simulink model "right_hand_rule"  (R2016a)
settings: Solver=FixedStepAuto  StartTime=0.0  StopTime=10.0  FixedStep=0.002  RelTol=1e-3
undefined symbols (not defined in the file or in its folder): exterm
libraries: simulink x1
settings Model: Creator=max  LastModifiedBy=max

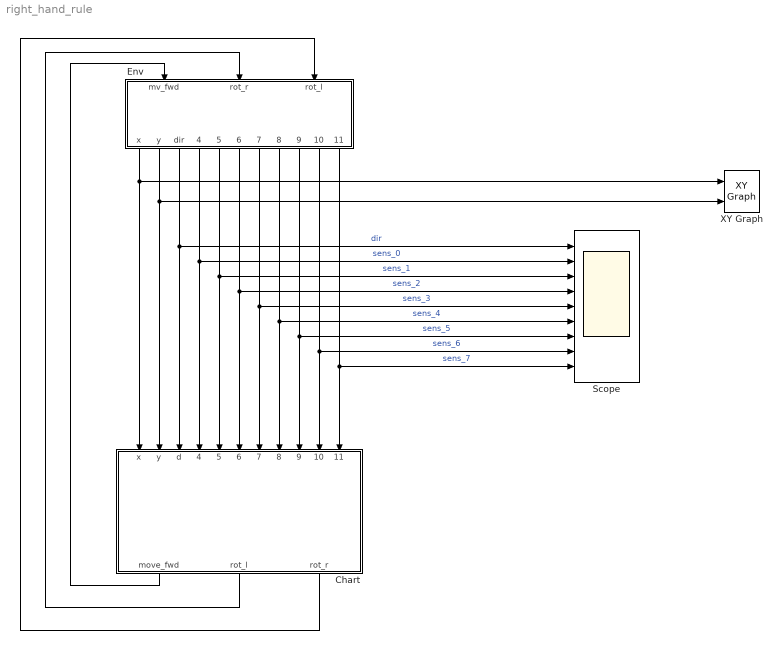
== system right_hand_rule ==
  Chart : Stateflow chart  TreatAsAtomicUnit=on
  Env : Subsystem
  Scope : Scope  NumInputPorts=9
  XY Graph : simulink/Sinks/XY Graph  xmin=-1  xmax=1  ymin=-1  ymax=1  st=-1
  wires:
  Chart/1(move_fwd) -> Env/1(mv_fwd)
  Chart/2(rot_l) -> Env/2(rot_r)
  Chart/3(rot_r) -> Env/3(rot_l)
  Env/1(x) -> Chart/1(x), XY Graph/1
  Env/4(sens_0) -> Chart/4(s_m150), Scope/2  "sens_0"
  Env/5(sens_1) -> Chart/5(s_m90), Scope/3  "sens_1"
  Env/6(sens_2) -> Chart/6(s_m45), Scope/4  "sens_2"
  Env/7(sens_3) -> Chart/7(s_m20), Scope/5  "sens_3"
  Env/8(sens_4) -> Chart/8(s_p20), Scope/6  "sens_4"
  Env/9(sens_5) -> Chart/9(s_p45), Scope/7  "sens_5"
  Env/10(sens_6) -> Chart/10(s_p90), Scope/8  "sens_6"
  Env/11(sens_7) -> Chart/11(s_p150), Scope/9  "sens_7"
  Env/2(y) -> Chart/2(y), XY Graph/2
  Env/3(dir) -> Chart/3(d), Scope/1  "dir"

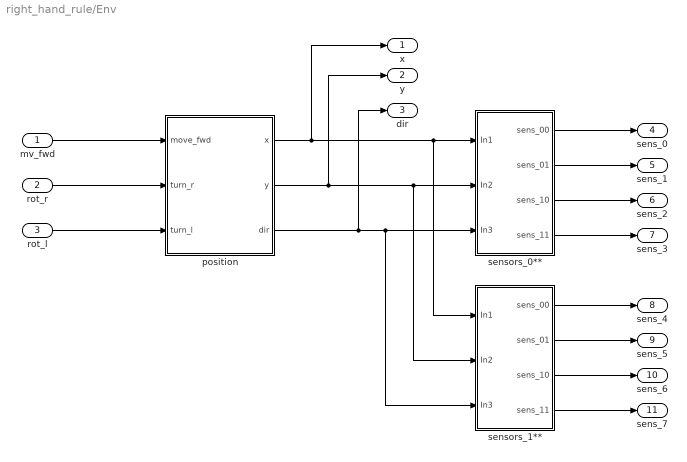
== system right_hand_rule/Env ==
  mv_fwd : Inport
  rot_r : Inport  Port=2
  rot_l : Inport  Port=3
  position : Subsystem
  sensors_0** : Subsystem
  sensors_1** : Subsystem
  x : Outport
  y : Outport  Port=2
  dir : Outport  Port=3
  sens_0 : Outport  Port=4
  sens_1 : Outport  Port=5
  sens_2 : Outport  Port=6
  sens_3 : Outport  Port=7
  sens_4 : Outport  Port=8
  sens_5 : Outport  Port=9
  sens_6 : Outport  Port=10
  sens_7 : Outport  Port=11
  wires:
  mv_fwd/1 -> position/1(move_fwd)
  rot_r/1 -> position/2(turn_r)
  rot_l/1 -> position/3(turn_l)
  sensors_0**/1(sens_00) -> sens_0/1
  sensors_0**/2(sens_01) -> sens_1/1
  sensors_0**/3(sens_10) -> sens_2/1
  sensors_0**/4(sens_11) -> sens_3/1
  position/1(x) -> x/1, sensors_1**/1(In1), sensors_0**/1(In1)
  position/2(y) -> sensors_1**/2(In2), sensors_0**/2(In2), y/1
  position/3(dir) -> dir/1, sensors_1**/3(In3), sensors_0**/3(In3)
  sensors_1**/1(sens_00) -> sens_4/1
  sensors_1**/2(sens_01) -> sens_5/1
  sensors_1**/3(sens_10) -> sens_6/1
  sensors_1**/4(sens_11) -> sens_7/1

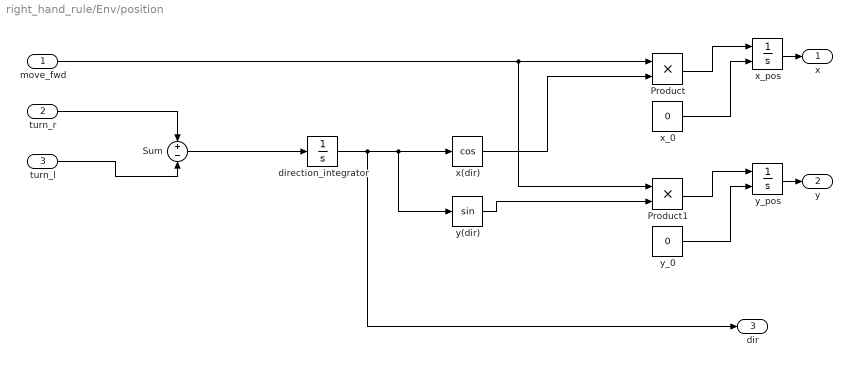
== system right_hand_rule/Env/position ==
  move_fwd : Inport
  turn_r : Inport  Port=2
  turn_l : Inport  Port=3
  Product : Product
  Product1 : Product
  Sum : Sum  Inputs=+-
  "direction_integrator " : Integrator
  x(dir) : Trigonometry  Operator=cos
  x_0 : Constant  Value=0
  x_pos : Integrator  InitialConditionSource=external  InitialCondition=exterm
  y(dir) : Trigonometry
  y_0 : Constant  Value=0
  y_pos : Integrator  InitialConditionSource=external  InitialCondition=exterm
  x : Outport
  y : Outport  Port=2
  dir : Outport  Port=3
  wires:
  turn_l/1 -> Sum/2
  Sum/1 -> "direction_integrator "/1
  turn_r/1 -> Sum/1
  y_pos/1 -> y/1
  x_0/1 -> x_pos/2
  x_pos/1 -> x/1
  x(dir)/1 -> Product/2
  Product/1 -> x_pos/1
  y(dir)/1 -> Product1/2
  Product1/1 -> y_pos/1
  move_fwd/1 -> Product1/1, Product/1
  y_0/1 -> y_pos/2
  "direction_integrator "/1 -> dir/1, y(dir)/1, x(dir)/1

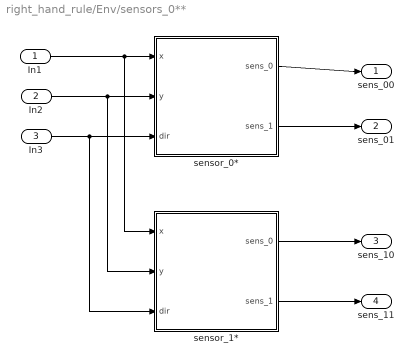
== system right_hand_rule/Env/sensors_0** ==
  In1 : Inport
  In2 : Inport  Port=2
  In3 : Inport  Port=3
  sensor_0* : Subsystem
  sensor_1* : Subsystem
  sens_00 : Outport
  sens_01 : Outport  Port=2
  sens_10 : Outport  Port=3
  sens_11 : Outport  Port=4
  wires:
  In3/1 -> sensor_1*/3(dir), sensor_0*/3(dir)
  sensor_1*/1(sens_0) -> sens_10/1
  sensor_1*/2(sens_1) -> sens_11/1
  sensor_0*/1(sens_0) -> sens_00/1
  sensor_0*/2(sens_1) -> sens_01/1
  In2/1 -> sensor_1*/2(y), sensor_0*/2(y)
  In1/1 -> sensor_1*/1(x), sensor_0*/1(x)

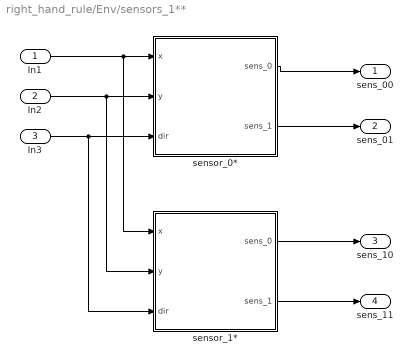
== system right_hand_rule/Env/sensors_1** ==
  In1 : Inport
  In2 : Inport  Port=2
  In3 : Inport  Port=3
  sensor_0* : Subsystem
  sensor_1* : Subsystem
  sens_00 : Outport
  sens_01 : Outport  Port=2
  sens_10 : Outport  Port=3
  sens_11 : Outport  Port=4
  wires:
  In3/1 -> sensor_1*/3(dir), sensor_0*/3(dir)
  sensor_1*/1(sens_0) -> sens_10/1
  sensor_1*/2(sens_1) -> sens_11/1
  sensor_0*/1(sens_0) -> sens_00/1
  sensor_0*/2(sens_1) -> sens_01/1
  In2/1 -> sensor_1*/2(y), sensor_0*/2(y)
  In1/1 -> sensor_1*/1(x), sensor_0*/1(x)

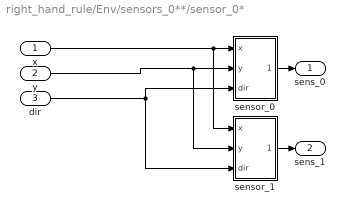
== system right_hand_rule/Env/sensors_0**/sensor_0* ==
  x : Inport
  y : Inport  Port=2
  dir : Inport  Port=3
  sensor_0 : Subsystem
  sensor_1 : Subsystem
  sens_0 : Outport
  sens_1 : Outport  Port=2
  wires:
  y/1 -> sensor_1/2(y), sensor_0/2(y)
  x/1 -> sensor_1/1(x), sensor_0/1(x)
  dir/1 -> sensor_1/3(dir), sensor_0/3(dir)
  sensor_0/1(dist) -> sens_0/1
  sensor_1/1(dist) -> sens_1/1

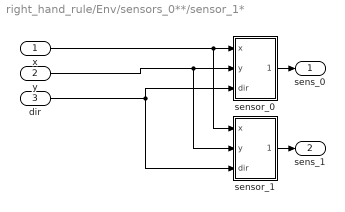
== system right_hand_rule/Env/sensors_0**/sensor_1* ==
  x : Inport
  y : Inport  Port=2
  dir : Inport  Port=3
  sensor_0 : Subsystem
  sensor_1 : Subsystem
  sens_0 : Outport
  sens_1 : Outport  Port=2
  wires:
  y/1 -> sensor_1/2(y), sensor_0/2(y)
  x/1 -> sensor_1/1(x), sensor_0/1(x)
  dir/1 -> sensor_1/3(dir), sensor_0/3(dir)
  sensor_0/1(dist) -> sens_0/1
  sensor_1/1(dist) -> sens_1/1

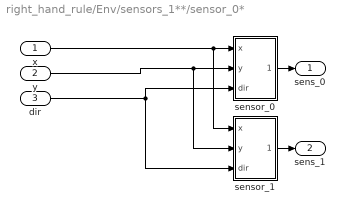
== system right_hand_rule/Env/sensors_1**/sensor_0* ==
  x : Inport
  y : Inport  Port=2
  dir : Inport  Port=3
  sensor_0 : Subsystem
  sensor_1 : Subsystem
  sens_0 : Outport
  sens_1 : Outport  Port=2
  wires:
  y/1 -> sensor_1/2(y), sensor_0/2(y)
  x/1 -> sensor_1/1(x), sensor_0/1(x)
  dir/1 -> sensor_1/3(dir), sensor_0/3(dir)
  sensor_0/1(dist) -> sens_0/1
  sensor_1/1(dist) -> sens_1/1

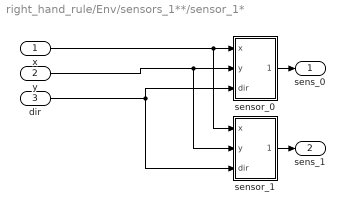
== system right_hand_rule/Env/sensors_1**/sensor_1* ==
  x : Inport
  y : Inport  Port=2
  dir : Inport  Port=3
  sensor_0 : Subsystem
  sensor_1 : Subsystem
  sens_0 : Outport
  sens_1 : Outport  Port=2
  wires:
  y/1 -> sensor_1/2(y), sensor_0/2(y)
  x/1 -> sensor_1/1(x), sensor_0/1(x)
  dir/1 -> sensor_1/3(dir), sensor_0/3(dir)
  sensor_0/1(dist) -> sens_0/1
  sensor_1/1(dist) -> sens_1/1

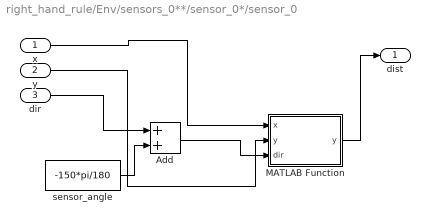
== system right_hand_rule/Env/sensors_0**/sensor_0*/sensor_0 ==
  x : Inport
  y : Inport  Port=2
  dir : Inport  Port=3
  Add : Sum
  MATLAB Function : MATLAB Function  TreatAsAtomicUnit=on
  sensor_angle : Constant  Value=-150*pi/180
  dist : Outport
  wires:
  sensor_angle/1 -> Add/2
  MATLAB Function/1(y) -> dist/1
  dir/1 -> Add/1
  Add/1 -> MATLAB Function/3(dir)
  x/1 -> MATLAB Function/1(x)
  y/1 -> MATLAB Function/2("y ")

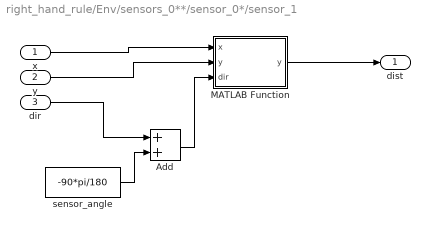
== system right_hand_rule/Env/sensors_0**/sensor_0*/sensor_1 ==
  x : Inport
  y : Inport  Port=2
  dir : Inport  Port=3
  Add : Sum
  MATLAB Function : MATLAB Function  TreatAsAtomicUnit=on
  sensor_angle : Constant  Value=-90*pi/180
  dist : Outport
  wires:
  sensor_angle/1 -> Add/2
  MATLAB Function/1(y) -> dist/1
  dir/1 -> Add/1
  Add/1 -> MATLAB Function/3(dir)
  x/1 -> MATLAB Function/1(x)
  y/1 -> MATLAB Function/2("y ")

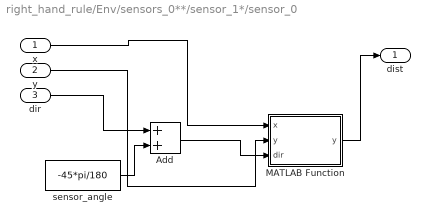
== system right_hand_rule/Env/sensors_0**/sensor_1*/sensor_0 ==
  x : Inport
  y : Inport  Port=2
  dir : Inport  Port=3
  Add : Sum
  MATLAB Function : MATLAB Function  TreatAsAtomicUnit=on
  sensor_angle : Constant  Value=-45*pi/180
  dist : Outport
  wires:
  sensor_angle/1 -> Add/2
  MATLAB Function/1(y) -> dist/1
  dir/1 -> Add/1
  Add/1 -> MATLAB Function/3(dir)
  x/1 -> MATLAB Function/1(x)
  y/1 -> MATLAB Function/2("y ")

== system right_hand_rule/Env/sensors_0**/sensor_1*/sensor_1 ==
  x : Inport
  y : Inport  Port=2
  dir : Inport  Port=3
  Add : Sum
  MATLAB Function : MATLAB Function  TreatAsAtomicUnit=on
  sensor_angle : Constant  Value=-20*pi/180
  dist : Outport
  wires:
  sensor_angle/1 -> Add/2
  MATLAB Function/1(y) -> dist/1
  dir/1 -> Add/1
  Add/1 -> MATLAB Function/3(dir)
  x/1 -> MATLAB Function/1(x)
  y/1 -> MATLAB Function/2("y ")

== system right_hand_rule/Env/sensors_1**/sensor_0*/sensor_0 ==
  x : Inport
  y : Inport  Port=2
  dir : Inport  Port=3
  Add : Sum
  MATLAB Function : MATLAB Function  TreatAsAtomicUnit=on
  sensor_angle : Constant  Value=20*pi/180
  dist : Outport
  wires:
  sensor_angle/1 -> Add/2
  MATLAB Function/1(y) -> dist/1
  dir/1 -> Add/1
  Add/1 -> MATLAB Function/3(dir)
  x/1 -> MATLAB Function/1(x)
  y/1 -> MATLAB Function/2("y ")

== system right_hand_rule/Env/sensors_1**/sensor_0*/sensor_1 ==
  x : Inport
  y : Inport  Port=2
  dir : Inport  Port=3
  Add : Sum
  MATLAB Function : MATLAB Function  TreatAsAtomicUnit=on
  sensor_angle : Constant  Value=45*pi/180
  dist : Outport
  wires:
  sensor_angle/1 -> Add/2
  MATLAB Function/1(y) -> dist/1
  dir/1 -> Add/1
  Add/1 -> MATLAB Function/3(dir)
  x/1 -> MATLAB Function/1(x)
  y/1 -> MATLAB Function/2("y ")

== system right_hand_rule/Env/sensors_1**/sensor_1*/sensor_0 ==
  x : Inport
  y : Inport  Port=2
  dir : Inport  Port=3
  Add : Sum
  MATLAB Function : MATLAB Function  TreatAsAtomicUnit=on
  sensor_angle : Constant  Value=90*pi/180
  dist : Outport
  wires:
  sensor_angle/1 -> Add/2
  MATLAB Function/1(y) -> dist/1
  dir/1 -> Add/1
  Add/1 -> MATLAB Function/3(dir)
  x/1 -> MATLAB Function/1(x)
  y/1 -> MATLAB Function/2("y ")

== system right_hand_rule/Env/sensors_1**/sensor_1*/sensor_1 ==
  x : Inport
  y : Inport  Port=2
  dir : Inport  Port=3
  Add : Sum
  MATLAB Function : MATLAB Function  TreatAsAtomicUnit=on
  sensor_angle : Constant  Value=150*pi/180
  dist : Outport
  wires:
  sensor_angle/1 -> Add/2
  MATLAB Function/1(y) -> dist/1
  dir/1 -> Add/1
  Add/1 -> MATLAB Function/3(dir)
  x/1 -> MATLAB Function/1(x)
  y/1 -> MATLAB Function/2("y ")

== matlab function right_hand_rule/Env/sensors_0**/sensor_0*/sensor_1/MATLAB Function ==
  data: x input; y output; y input; dir input
function y = fcn(x,y,dir)
y = intersectQuarterPlane(x,y,dir);

== matlab function right_hand_rule/Env/sensors_0**/sensor_0*/sensor_0/MATLAB Function ==
  data: x input; y output; y input; dir input
function y = fcn(x,y,dir)
y = intersectQuarterPlane(x,y,dir);

== stateflow chart right_hand_rule/Chart ==
  state claustrophobia
    % known: have -20, -45, -90
    entry:
    move_fwd = 0;
    rot_l = 1;
    rot_r = 0;
  state avoidCollision
    % known: have -20, -45
    entry:
    move_fwd = 0;
    rot_l = 1;
    rot_r = 0;
  state orientToWall
    % known: have -20
    % rotate left until we "touch the wall"
    entry:
    move_fwd = 1;
    rot_r = 0;
    rot_l = 0;
  state findWall
    entry:
    move_fwd=1;
    rot_l = d + 0;
    rot_r = 0;
  state follow
    % known: have -45, -90
    entry:
    move_fwd = 1;
    rot_l = 0;
    rot_r = 0;
  state stayClose
    % known: have -90, NOT have -45
    entry:
    move_fwd = 0;
    rot_l = 0;
    rot_r = 1;
  (default) -> findWall
  orientToWall -> avoidCollision : [s_m45 <= sens_tol]
  avoidCollision -> claustrophobia [order 2] : [s_m90 <= sens_tol]
  avoidCollision -> orientToWall [order 1] : [s_m45 > sens_tol]
  findWall -> orientToWall : [s_m20 <= sens_tol]
  stayClose -> orientToWall : [s_m20 <= sens_tol && after(90*(pi/180)/rot_per_sec, sec)]
  follow -> claustrophobia [order 1] : [s_m20 <= sens_tol]
  claustrophobia -> follow : [s_m20 > sens_tol]
  follow -> stayClose [order 2] : [s_m45 > sens_tol]
  data: x input; y input; d input; move_fwd output; rot_l output; rot_r output; s_m150 input; s_m90 input; s_m45 input; s_m20 input; s_p20 input; s_p45 input; s_p90 input; s_p150 input; sens_tol constant double; rot_per_sec constant double =1

== matlab function right_hand_rule/Env/sensors_0**/sensor_1*/sensor_0/MATLAB Function ==
  data: x input; y output; y input; dir input
function y = fcn(x,y,dir)
y = intersectQuarterPlane(x,y,dir);

== matlab function right_hand_rule/Env/sensors_0**/sensor_1*/sensor_1/MATLAB Function ==
  data: x input; y output; y input; dir input
function y = fcn(x,y,dir)
y = intersectQuarterPlane(x,y,dir);

== matlab function right_hand_rule/Env/sensors_1**/sensor_0*/sensor_0/MATLAB Function ==
  data: x input; y output; y input; dir input
function y = fcn(x,y,dir)
y = intersectQuarterPlane(x,y,dir);

== matlab function right_hand_rule/Env/sensors_1**/sensor_0*/sensor_1/MATLAB Function ==
  data: x input; y output; y input; dir input
function y = fcn(x,y,dir)
y = intersectQuarterPlane(x,y,dir);

== matlab function right_hand_rule/Env/sensors_1**/sensor_1*/sensor_0/MATLAB Function ==
  data: x input; y output; y input; dir input
function y = fcn(x,y,dir)
y = intersectQuarterPlane(x,y,dir);

== matlab function right_hand_rule/Env/sensors_1**/sensor_1*/sensor_1/MATLAB Function ==
  data: x input; y output; y input; dir input
function y = fcn(x,y,dir)
y = intersectQuarterPlane(x,y,dir);
